simulink model "Dual_Path_logic"  (R2025b)
settings: Solver=FixedStepAuto  StartTime=0.0  StopTime=10.0  RelTol=1e-3
settings Model: Creator=strog  LastModifiedBy=strog
settings OptimizationCC: DefaultParameterBehavior=Inlined  UseDivisionForNetSlopeComputation=on  GainParamInheritBuiltInType=on  UseFloatMulNetSlope=on  InlineInvariantSignals=on  PassReuseOutputArgsAs=Individual arguments  ZeroExternalMemoryAtStartup=off  ZeroInternalMemoryAtStartup=off  NoFixptDivByZeroProtection=on  EfficientFloat2IntCast=on  LifeSpan=1  OptimizeBlockOrder=speed  DifferentSizesBufferReuse=on  EfficientTunableParamExpr=on
settings DebuggingCC: ParameterTunabilityLossMsg=error
settings HardwareCC: ProdLongLongMode=on  ProdHWDeviceType=AMD->x86-64 (Windows64)
settings SFSimCC: MATLABDynamicMemAlloc=off
settings RTWCC: SystemTargetFile=ert.tlc  TemplateMakefile=ert_default_tmf  Description=Embedded Coder
settings CodeAppCC: ForceParamTrailComments=on  IgnoreCustomStorageClasses=off  OperatorAnnotations=on  SimulinkDataObjDesc=on  SFDataObjDesc=on  CustomSymbolStrGlobalVar=rt$N$M  CustomSymbolStrType=$N$M  CustomSymbolStrFcn=$N$M$F  CustomSymbolStrMacro=$N$M  InsertBlockDesc=on
settings ERTTargetCC: ERTCustomFileTemplate=example_file_process.tlc  ERTFilePackagingFormat=CompactWithDataFile  TargetLangStandard=C99 (ISO)  GenerateSampleERTMain=on  IncludeMdlTerminateFcn=off  CombineSignalStateStructs=on  SupportAbsoluteTime=off  SupportComplex=off  SupportContinuousTime=on  SupportNonInlinedSFcns=on

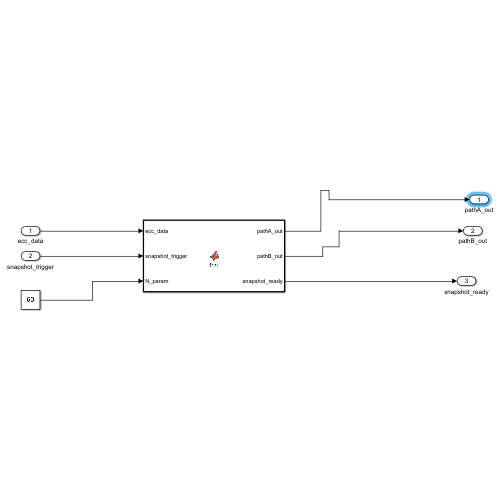
[thumbnail: Simulink's stored preview of the top-level diagram]
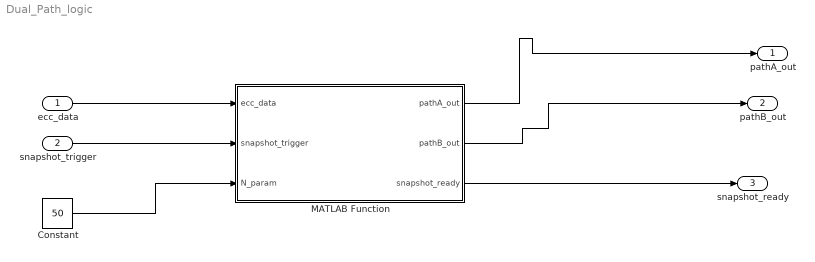
== system Dual_Path_logic ==
  ecc_data : Inport
  snapshot_trigger : Inport  Port=2
  Constant : Constant  Value=50
  MATLAB Function : MATLAB Function  TreatAsAtomicUnit=on
  pathA_out : Outport  PortDimensions=1
  pathB_out : Outport  Port=2  PortDimensions=100
  snapshot_ready : Outport  Port=3
  wires:
  MATLAB Function/2(pathB_out) -> pathB_out/1
  MATLAB Function/3(snapshot_ready) -> snapshot_ready/1
  Constant/1 -> MATLAB Function/3(N_param)
  snapshot_trigger/1 -> MATLAB Function/2(snapshot_trigger)
  MATLAB Function/1(pathA_out) -> pathA_out/1
  ecc_data/1 -> MATLAB Function/1(ecc_data)

== matlab function Dual_Path_logic/MATLAB Function ==
  data: ecc_data input; pathA_out output size=1; snapshot_trigger input; N_param input; pathB_out output size=100; snapshot_ready output
function [pathA_out, pathB_out, snapshot_ready] = fcn(ecc_data, snapshot_trigger, N_param)
% #codegen

length_N = 50; 
total_window = length_N * 2;

persistent ring_buffer;    
persistent sample_counter; 
persistent hold_counter;   
persistent is_recording;   
persistent final_snapshot; 

if isempty(ring_buffer)
    ring_buffer = zeros(total_window, 1); % Вектор-столбец
    sample_counter = 0;
    hold_counter = 0;
    is_recording = false;
    final_snapshot = zeros(total_window, 1);
end

%% ==================== PATH A ====================
sample_counter = sample_counter + 1;
if sample_counter >= 1000
    pathA_out = ecc_data;
    sample_counter = 0;
else
    pathA_out = 0.0; 
end

%% ==================== PATH B ====================
% Сдвиг через точку с запятой для вертикального вектора
ring_buffer = [ring_buffer(2:end); ecc_data];

snapshot_ready = false;

if snapshot_trigger && ~is_recording
    is_recording = true;
    hold_counter = 0;
end

if is_recording
    hold_counter = hold_counter + 1;
    if hold_counter >= length_N
        final_snapshot = ring_buffer; 
        is_recording = false;         
        hold_counter = 0;
        snapshot_ready = true;        
    end
end

pathB_out = final_snapshot;
